simulink model "FG_RealTime_EP_P1"  (R2017b)
settings: Solver=FixedStepDiscrete  StartTime=0.0  StopTime=inf  FixedStep=UserParams.SampleTime  RelTol=1e-3  EnableMultiTasking=on
InitFcn:
  | isSim = 0;
  | PreFunctions.CustomInitFcn;
model workspace (MATLAB code in the model file + MAT data in the model file):
  isSim = 0
  A_lpf_velocity_IMU = 0.0790363191017
  A_lpf_velocity_joint = 0.0790363191017
  B1_lpf_velocity_IMU = -1.56224419787
  B1_lpf_velocity_joint = -1.56224419787
  B2_lpf_velocity_IMU = 0.641280516968
  B2_lpf_velocity_joint = 0.641280516968
  Data.hd = [0; 0; 0; 0; 0; 0; 0; 0; 0; 0]
  Data.dhd = [0; 0; 0; 0; 0; 0; 0; 0; 0; 0]
  Data.h0 = [0; 0; 0; 0; 0; 0; 0; 0; 0; 0]
  Data.dh0 = [0; 0; 0; 0; 0; 0; 0; 0; 0; 0]
  Data.hd_fix = [0; 0; 0; 0; 0; 0; 0; 0; 0; 0]
  Data.dhd_fix = [0; 0; 0; 0; 0; 0; 0; 0; 0; 0]
  Data.h0_fix = [0; 0; 0; 0; 0; 0; 0; 0; 0; 0]
  Data.dh0_fix = [0; 0; 0; 0; 0; 0; 0; 0; 0; 0]
  Data.hd_joint = [0; 0; 0; 0; 0; 0; 0; 0; 0; 0]
  Data.dhd_joint = [0; 0; 0; 0; 0; 0; 0; 0; 0; 0]
  Data.h0_joint = [0; 0; 0; 0; 0; 0; 0; 0; 0; 0]
  Data.dh0_joint = [0; 0; 0; 0; 0; 0; 0; 0; 0; 0]
  Data.y = [0; 0; 0; 0; 0; 0; 0; 0; 0; 0]
  Data.dy = [0; 0; 0; 0; 0; 0; 0; 0; 0; 0]
  Data.y_joint = [0; 0; 0; 0; 0; 0; 0; 0; 0; 0]
  Data.dy_joint = [0; 0; 0; 0; 0; 0; 0; 0; 0; 0]
  Data.y1_joint = 0
  Data.y2_joint = 0
  Data.y3_joint = 0
  Data.y4_joint = 0
  Data.y5_joint = 0
  Data.y6_joint = 0
  Data.y7_joint = 0
  Data.y8_joint = 0
  Data.y9_joint = 0
  Data.y10_joint = 0
  Data.y_knee = [0; 0]
  Data.dy_knee = [0; 0]
  Data.LLd = 0
  Data.dLLd = 0
  Data.qKnee_d = 0
  Data.dqKnee_d = 0
  Data.qknee_d_L = 0
  Data.qknee_d_R = 0
  Data.left_tune = 0
  Data.right_tune = 0
  Data.LL0_R = 0
  Data.LL0_L = 0
  Data.y_output = [0; 0; 0; 0]
  Data.dy_output = [0; 0; 0; 0]
  Data.u_output = [0; 0; 0; 0]
  Data.lateral_mid_p = 0
  Data.lateral_mid_v = 0
  Data.LL_des_fil = 0
  Data.test = 0
  Data.task = 0
  Data.t = 0
  Data.q = [0; 0; 0; 0; 0; 0; 0; 0; 0; 0; 0; 0; 0; 0; 0; 0; 0; 0; 0; 0; 0; 0; 0; 0; 0; 0]
  Data.dq = [0; 0; 0; 0; 0; 0; 0; 0; 0; 0; 0; 0; 0; 0; 0; 0; 0; 0; 0; 0; 0; 0; 0; 0; 0; 0]
  Data.u = [0; 0; 0; 0; 0; 0; 0; 0; 0; 0]
  Data.u_sat = [0; 0; 0; 0; 0; 0; 0; 0; 0; 0]
  Data.u_fil = [0; 0; 0; 0; 0; 0; 0; 0; 0; 0]
  Data.stanceLeg = 0
  Data.s_sw = 0
  Data.s_st = 0
  Data.s = 0
  Data.ds = 0
  Data.encoder_fil = [0; 0; 0; 0; 0; 0; 0; 0; 0; 0; 0; 0; 0; 0]
  Data.d_torso_angle_fil = [0; 0; 0]
  Data.tp_last = 0
  Data.avg_v_last_1 = 0
  Data.avg_v_last_2 = 0
  Data.theta = 0
  Data.dtheta = 0
  Data.theta_d = 0
  Data.dtheta_d = 0
  Data.GRF = [0; 0]
  Data.t0 = 0
  Data.Switch = 0
  Data.spring_force_R = [0; 0]
  Data.spring_force_L = [0; 0]
  Data.torso_angle = [0; 0; 0]
  Data.d_torso_angle = [0; 0; 0]
  Data.id_torso_angle = [0; 0; 0]
  Data.dd_torso_angle = [0; 0; 0]
  Data.torso_position = [0; 0; 0]
  Data.torso_velocity = [0; 0; 0]
  Data.torso_velocity_fil = [0; 0; 0]
  Data.torso_vx = 0
  Data.torso_vy = 0
  Data.torso_vz = 0
  Data.torso_vx_fil = 0
  Data.torso_vy_fil = 0
  Data.torso_vz_fil = 0
  Data.torso_vx_b = 0
  Data.torso_vy_b = 0
  Data.torso_vz_b = 0
  Data.torso_vx_b_fil = 0
  Data.torso_vy_b_fil = 0
  Data.torso_vz_b_fil = 0
  Data.tg_velocity_x = 0
  Data.com_pos = [0; 0; 0]
  Data.com_vel = [0; 0; 0]
  Data.com_vel_x = 0
  Data.com_vel_y = 0
  Data.com_vel_z = 0
  Data.com_vel_x_fil = 0
  Data.com_vel_y_fil = 0
  Data.com_vel_z_fil = 0
  Data.com_pos_x_fil = 0
  Data.com_pos_y_fil = 0
  Data.com_pos_z_fil = 0
  Data.com_pos_fil = [0; 0; 0]
  Data.torso_vx_test = 0
  Data.torso_vy_test = 0
  Data.torso_vz_test = 0
  Data.torso_vx_b_test = 0
  Data.torso_vy_b_test = 0
  Data.torso_vz_b_test = 0
  Data.torso_vx_test_2 = 0
  Data.torso_vy_test_2 = 0
  Data.torso_vz_test_2 = 0
  Data.torso_vx_b_test_2 = 0
  Data.torso_vy_b_test_2 = 0
  Data.torso_vz_b_test_2 = 0
  Data.torso_vx_fil_test = 0
  Data.torso_vy_fil_test = 0
  Data.torso_vz_fil_test = 0
  Data.torso_vx_b_fil_test = 0
  Data.torso_vy_b_fil_test = 0
  Data.torso_vz_b_fil_test = 0
  Data.dqy_b_avg_1 = 0
  Data.l_abduction_vx = 0
  Data.l_abduction_vy = 0
  Data.l_abduction_vz = 0
  Data.l_foot_vx = 0
  Data.l_foot_vy = 0
  Data.l_foot_vz = 0
  Data.l_foot_vx_b = 0
  Data.l_foot_vy_b = 0
  Data.l_foot_vz_b = 0
  Data.r_foot_v = [0; 0; 0]
  Data.l_foot_v = [0; 0; 0]
  Data.r_foot_p = [0; 0; 0]
  Data.l_foot_p = [0; 0; 0]
  Data.s_LR = [0; 0]
  Data.orient = 0
  Data.d_orient_test = 0
  Data.d_orient = 0
  Data.step_end_dx_fil_seq = [0; 0; 0]
  Data.step_end_dy_fil_seq = [0; 0; 0]
  Data.q_abduction_R = 0
  Data.q_rotation_R = 0
  Data.q_thigh_R = 0
  Data.q_thigh_knee_R = 0
  Data.q_knee_shin_R = 0
  Data.q_thigh_shin_R = 0
  Data.q_shin_tarsus_R = 0
  Data.q_toe_R = 0
  Data.q_abduction_L = 0
  Data.q_rotation_L = 0
  Data.q_thigh_L = 0
  Data.q_thigh_knee_L = 0
  Data.q_knee_shin_L = 0
  Data.q_thigh_shin_L = 0
  Data.q_shin_tarsus_L = 0
  Data.q_toe_L = 0
  Data.dq_abduction_R = 0
  Data.dq_rotation_R = 0
  Data.dq_thigh_R = 0
  Data.dq_thigh_knee_R = 0
  Data.dq_knee_shin_R = 0
  Data.dq_thigh_shin_R = 0
  Data.dq_shin_tarsus_R = 0
  Data.dq_toe_R = 0
  Data.dq_abduction_L = 0
  Data.dq_rotation_L = 0
  Data.dq_thigh_L = 0
  Data.dq_thigh_knee_L = 0
  Data.dq_knee_shin_L = 0
  Data.dq_thigh_shin_L = 0
  Data.dq_shin_tarsus_L = 0
  Data.dq_toe_L = 0
  Data.qall = [0; 0; 0; 0; 0; 0; 0; 0; 0; 0; 0; 0; 0; 0; 0; 0; 0; 0; 0; 0]
  Data.dqall = [0; 0; 0; 0; 0; 0; 0; 0; 0; 0; 0; 0; 0; 0; 0; 0; 0; 0; 0; 0]
  Data.qq = [0; 0; 0; 0]
  Data.qaR = [0; 0; 0; 0; 0]
  Data.qjR = [0; 0]
  Data.qsR = [0; 0]
  Data.qaL = [0; 0; 0; 0; 0]
  Data.qjL = [0; 0]
  Data.qsL = [0; 0]
  Data.dqq = [0; 0; 0]
  Data.dqaR = [0; 0; 0; 0; 0]
  Data.dqjR = [0; 0]
  Data.dqsR = [0; 0]
  Data.dqaL = [0; 0; 0; 0; 0]
  Data.dqjL = [0; 0]
  Data.dqsL = [0; 0]
  Data.u_P = [0; 0; 0; 0; 0; 0; 0; 0; 0; 0]
  Data.u_D = [0; 0; 0; 0; 0; 0; 0; 0; 0; 0]
  Data.hd_original = [0; 0; 0; 0; 0; 0; 0; 0; 0; 0]
  Data.u_CP_stance_knee = 0
  Data.e_CP_stance_knee = 0
  Data.u_OT_stance_knee = 0
  Data.u_CP_stance_hip_pitch = 0
  Data.e_CP_stance_hip_pitch = 0
  Data.u_OT_stance_hip_pitch = 0
  Data.u_CP_stance_abduction = 0
  Data.e_CP_stance_abduction = 0
  Data.u_OT_stance_abduction = 0
  Data.computer_time = 0
  Data.Torque_CP = [0; 0; 0; 0; 0; 0; 0; 0; 0; 0]
  Data.Error_CP = [0; 0; 0; 0; 0; 0; 0; 0; 0; 0]
  Data.RadioChannel = [0; 0; 0; 0; 0; 0; 0; 0; 0; 0; 0; 0; 0; 0; 0; 0]
  Data.lateral_ftpl = 0
  Data.I_Vel = [0; 0; 0]
  Data.EKF_v = [0; 0; 0]
  Data.EKF_q = [0; 0; 0; 0; 0; 0; 0; 0; 0; 0; 0; 0; 0; 0; 0; 0; 0; 0; 0; 0]
  Data.EKF_dq = [0; 0; 0; 0; 0; 0; 0; 0; 0; 0; 0; 0; 0; 0; 0; 0; 0; 0; 0; 0]
  UserParams.SampleTime = 0.0005
  c_CP_StanceAbdu = [0 70 40 60 0]
  c_CP_StanceKnee = [60 280 -40 -20 20]
  c_CP_SwingAbdu = [-5 -8 10 15 -5]
  c_CP_SwingKnee = [0 0 0 0 0]
  c_Gamma_st_abu = 120
  c_Gamma_st_hip = 0.5
  c_Gamma_st_knee = 150
  c_Gamma_sw_abu = 120
  c_Gamma_sw_hip = 0.1
  c_Gamma_sw_knee = 1.5
  c_Kd_abduction = 10
  c_Kd_abduction_stand = 4
  c_Kd_knee = 15
  c_Kd_knee_stand = 20
  c_Kd_lateral_stand = 0.025
  c_Kd_pitch = 40
  c_Kd_roll = 30
  c_Kd_rotation = 10
  c_Kd_rotation_stand = 4
  c_Kd_thigh = 15
  c_Kd_thigh_stand = 10
  c_Kd_toe = 2
  c_Kd_toe_stand = 80
  c_Kd_yaw = 4
  c_Kfl_d = 0.5
  c_Kfl_p = 0.25
  c_Kfs_d = 0.08
  c_Kfs_p = 0.05
  c_Kp_abduction = 600
  c_Kp_abduction_stand = 400
  c_Kp_knee = 500
  c_Kp_knee_stand = 500
  c_Kp_lateral_stand = 2
  c_Kp_pitch = 800
  c_Kp_roll = 500
  c_Kp_rotation = 800
  c_Kp_rotation_stand = 200
  c_Kp_thigh = 500
  c_Kp_thigh_stand = 200
  c_Kp_toe = 10
  c_Kp_toe_stand = 600
  c_Kp_yaw = 200
  c_abduction_inward_gain = 1
  c_com_bp = 0.05
  c_fil_para_2 = 0.02
  c_fil_para_3 = 0.02
  c_fil_para_4 = 0.001
  c_fil_para_5 = 0.02
  c_fil_para_x = 0.002
  c_fil_para_y = 0.002
  c_fil_vel_offset = 0
  c_final_st_abduction = 0.05
  c_final_sw_abduction = 0.15
  c_force_step_end_s = 1
  c_init_lateral_velocity = 0.1
  c_joint_filter_choice = 1
  c_lateral_offset_exp = 0
  c_lateral_velocity_weight = 1
  c_pre_final_sw_abduction = -0.01
  c_sagittal_offset_exp = 0
  c_sagittal_speed = 0
  c_shift_distance = 0.03
  c_shift_time = 0.4
  c_stance_thre_lb = 100
  c_stance_thre_ub = 200
  c_stand_offset_exp = 0
  c_standing_switch_time = 0.4
  c_toe_tilt_angle = 0
  c_turning_offset_exp = 0
  c_u_abduction_cp = 40
  c_u_abduction_swing_cp = 14
  c_u_knee_cp = 120
  c_u_thigh_cp = -15
  cassieDataBusInfo.block = []
  cassieDataBusInfo.busName = 'slBus38'
  fcut_velocity_IMU = 628.318530718
  fcut_velocity_joint = 628.318530718
  lpf_damping = 0.707106781187
  sample_time = 0.0005
  other statements: PreFunctions.CustomInitFcn;
libraries: FG_Controller_Library x1
settings Model: TunableVars=c_CP_StanceAbdu,c_CP_StanceKnee,c_CP_SwingAbdu,c_CP_SwingKnee,c_Gamma_knee,c_Gamma_st_abu,c_Gamma_st_hip,c_Gamma_st_knee,c_Gamma_sw_abu,c_Gamma_sw_hip,c_Gamma_sw_knee,c_Kd_abduction,c_Kd_abduction_stand,c_Kd_knee,c_Kd_knee_stand,c_Kd_lateral_stand,c_Kd_pitch,c_Kd_roll,c_Kd_rotation,c_Kd_rotation_stand,c_Kd_thigh,c_Kd_thigh_stand,c_Kd_toe,c_Kd_toe_stand,c_Kd_yaw,c_Kfl_d,c_Kfl_p,c_Kfs_d,c_Kfs_p,c_Kp_abduction,c_Kp_abduction_stand,c_Kp_knee,c_Kp_knee_stand,c_Kp_lateral_stand,c_Kp_pitch,c_Kp_roll,c_Kp_rotation,c_Kp_rotation_stand,c_Kp_thigh,c_Kp_thigh_stand,c_Kp_toe,c_Kp_toe_stand,c_Kp_yaw,c_abduction_inward_gain,c_com_bp,c_fil_para_2,c_fil_para_3,c_fil_para_4,c_fil_para_5,c_fil_para_x,c_fil_para_y,c_fil_vel_offset,c_final_st_abduction,c_final_sw_abduction,c_force_step_end_s,c_init_lateral_velocity,c_joint_filter_choice,c_lateral_offset_exp,c_lateral_velocity_weight,c_pre_final_sw_abduction,c_sagittal_offset_exp,c_sagittal_speed,c_shift_distance,c_shift_time,c_stance_thre_lb,c_stance_thre_ub,c_stand_offset_exp,c_standing_switch_time,c_toe_tilt_angle,c_turning_offset_exp,c_u_abduction_cp,c_u_abduction_swing_cp,c_u_knee_cp,c_u_thigh_cp  TunableVarsStorageClass=Auto,Auto,Auto,Auto,Auto,Auto,Auto,Auto,Auto,Auto,Auto,Auto,Auto,Auto,Auto,Auto,Auto,Auto,Auto,Auto,Auto,Auto,Auto,Auto,Auto,Auto,Auto,Auto,Auto,Auto,Auto,Auto,Auto,Auto,Auto,Auto,Auto,Auto,Auto,Auto,Auto,Auto,Auto,Auto,Auto,Auto,Auto,Auto,Auto,Auto,Auto,Auto,Auto,Auto,Auto,Auto,Auto,Auto,Auto,Auto,Auto,Auto,Auto,Auto,Auto,Auto,Auto,Auto,Auto,Auto,Auto,Auto,Auto,Auto  TunableVarsTypeQualifier=,,,,,,,,,,,,,,,,,,,,,,,,,,,,,,,,,,,,,,,,,,,,,,,,,,,,,,,,,,,,,,,,,,,,,,,,,  Creator=robot  LastModifiedBy=RoahmLab
settings SolverCC: ConcurrentTasks=on
settings DataIOCC: SaveFormat=Array  SaveOutput=off  SignalLogging=off  DSMLogging=off  VisualizeSimOutput=off  SaveTime=off
settings OptimizationCC: LifeSpan=inf  SimCompilerOptimization=on  AccelVerboseBuild=on
settings DebuggingCC: AllowSymbolicDim=off  SFUnexpectedBacktrackingDiag=warning  SFNoUnconditionalDefaultTransitionDiag=warning  SFExecutionAtInitializationDiag=none
settings HardwareCC: ProdBitPerPointer=32  ProdBitPerSizeT=32  ProdBitPerPtrDiffT=32  ProdLargestAtomicFloat=None  ProdWordSize=32  ProdLongLongMode=on  ProdHWDeviceType=Generic->32-bit x86 compatible
settings ModelReferenceCC: ParallelModelReferenceMATLABWorkerInit=Copy Base Workspace  PropagateSignalLabelsOutOfModel=off
settings SFSimCC: SimUserIncludeDirs=D:\Graduate\robots\Cassie\GitHub\Cassie_Controller_V3_Yukai\Controllers\Flatground\utils\funcs\kin  SFSimEcho=off
settings SFSimCC: SimUserSources=|
  | ComPosition_src.c
  | ComVelocity_src.c
  | J_LeftToeBottomBack_src.c
  | J_LeftToeBottomFront_src.c
  | J_LeftToeBottom_src.c
  | J_LeftToeJoint_src.c
  | J_RightToeBottomBack_src.c
  | J_RightToeBottomFront_src.c
  | J_RightToeBottom_src.c
  | J_RightToeJoint_src.c
  | LeftToeBottomBack_src.c
  | LeftToeBottomFront_src.c
  | LeftToeBottom_src.c
  | LeftToeJoint_src.c
  | RightToeBottomBack_src.c
  | RightToeBottomFront_src.c
  | RightToeBottom_src.c
  | RightToeJoint_src.c
settings RTWCC: SystemTargetFile=slrt.tlc  TLCOptions=-axPCMaxOverloads=1000000000 -axPCMaxOverloadLen=1000000000  TemplateMakefile=slrt_default_tmf  Description=Simulink Real-Time  RTWUseSimCustomCode=on  CustomInclude=D:\Graduate\robots\Cassie\GitHub\Cassie_Controller_V3_Yukai\Controllers\Flatground\utils\funcs\kin  CodeExecutionProfiling=on  CodeProfilingSaveOptions=AllData  CodeProfilingInstrumentation=on  RTWCompilerOptimization=on
settings RTWCC: CustomSource=|
  | ComPosition_src.c
  | ComVelocity_src.c
  | J_LeftToeBottomBack_src.c
  | J_LeftToeBottomFront_src.c
  | J_LeftToeBottom_src.c
  | J_LeftToeJoint_src.c
  | J_RightToeBottomBack_src.c
  | J_RightToeBottomFront_src.c
  | J_RightToeBottom_src.c
  | J_RightToeJoint_src.c
  | LeftToeBottomBack_src.c
  | LeftToeBottomFront_src.c
  | LeftToeBottom_src.c
  | LeftToeJoint_src.c
  | RightToeBottomBack_src.c
  | RightToeBottomFront_src.c
  | RightToeBottom_src.c
  | RightToeJoint_src.c
settings CodeAppCC: GenerateComments=off  MaxIdLength=128  SimulinkBlockComments=off
settings ConfigComp: CovMetricSettings=dw  CovHtmlReporting=on  CovSaveCumulativeToWorkspaceVar=on  CovSaveSingleToWorkspaceVar=on  CovExternalEMLEnable=off

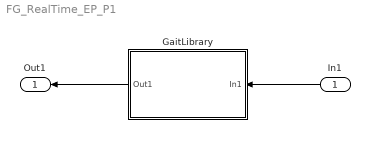
== system FG_RealTime_EP_P1 ==
  In1 : Inport
  GaitLibrary : Subsystem
  Out1 : Outport  OutDataTypeStr=Bus: cassieGLDataBus  BusOutputAsStruct=on
  wires:
  In1/1 -> GaitLibrary/1(In1)
  GaitLibrary/1(Out1) -> Out1/1

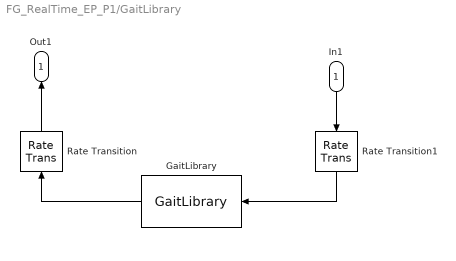
== system FG_RealTime_EP_P1/GaitLibrary ==
  In1 : Inport
  GaitLibrary : FG_Controller_Library/GaitLibrary
  Rate Transition : RateTransition  Deterministic=off  OutPortSampleTime=UserParams.SampleTime
  Rate Transition1 : RateTransition  Deterministic=off  OutPortSampleTime=0.01
  Out1 : Outport
  wires:
  Rate Transition/1 -> Out1/1
  In1/1 -> Rate Transition1/1
  Rate Transition1/1 -> GaitLibrary/1
  GaitLibrary/1 -> Rate Transition/1
